simulink model "observer_DT_simulink"  (R2022b)
settings: Solver=VariableStepAuto  StartTime=0.0  StopTime=10.0  RelTol=1e-3
undefined symbols (not defined in the file): Ahat, amplitude, Bhat, C_DT, Chat, D_DT, Dhat, freq, initpha, sys_DT, Ts, x0, xhat0
settings Model: Creator=tpjch  LastModifiedBy=xuchen

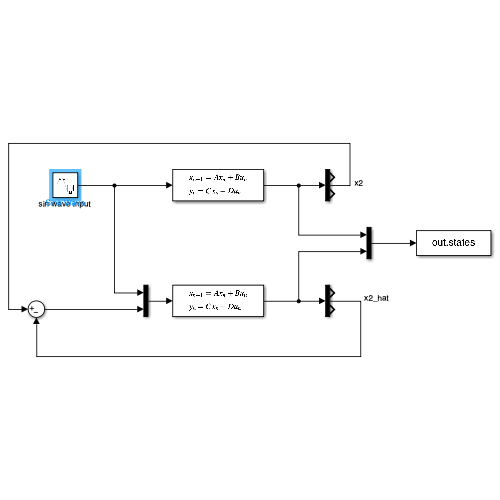
[thumbnail: Simulink's stored preview of the top-level diagram]
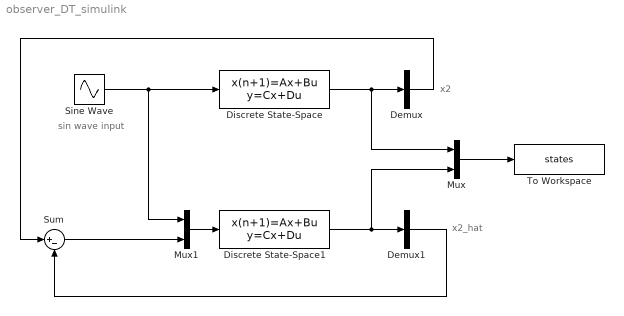
== system observer_DT_simulink ==
  note: x2
  note: x2_hat
  note: sin wave input
  Demux : Demux  Outputs=3
  Demux1 : Demux  Outputs=3
  Discrete State-Space : DiscreteStateSpace  A=sys_DT.A  B=sys_DT.B  C=C_DT  D=D_DT  InitialCondition=x0  SampleTime=Ts
  Discrete State-Space1 : DiscreteStateSpace  A=Ahat  B=Bhat  C=Chat  D=Dhat  InitialCondition=xhat0  SampleTime=Ts
  Mux : Mux  Inputs=2
  Mux1 : Mux  Inputs=2
  Sine Wave : Sin  Amplitude=amplitude  Frequency=freq  Phase=initpha  SampleTime=Ts
  Sum : Sum  Inputs=|+-
  To Workspace : ToWorkspace  VariableName=states  SaveFormat=Timeseries  SampleTime=-1
  wires:
  Discrete State-Space/1 -> Demux/1, Mux/1
  Mux/1 -> To Workspace/1
  Discrete State-Space1/1 -> Demux1/1, Mux/2
  Sine Wave/1 -> Discrete State-Space/1, Mux1/1
  Mux1/1 -> Discrete State-Space1/1
  Sum/1 -> Mux1/2
  Demux1/2 -> Sum/2
  Demux/2 -> Sum/1
